simulink model "sampleModel123"  (Simulink 9.1)
settings: Solver=VariableStepAuto  StartTime=0.0  StopTime=10.0  RelTol=1e-3
undefined symbols (not defined in the file): DiscIntNeverNeededParam, Newton, Raphson
libraries: simulink x12
settings Model: SuppressorTable="22 serialization::archive 11 0 6 0 0 1 8 0 0 0 0 6 0 0 1 0 22 sampleModel123/cfblk32 0 6 0 0 2 8 0 0 0 0 6 41 Simulink:DataType:WarningOverFlowDetected 0 0 0 6 0  0  0 0 0 0 8 20160523 0 0 0 10 57 55 0 1 40 SimulinkFixedPoint:util:Overflowoccurred 0 0 0  0  8 20160523 0 10 57 55 0 1"  Creator=DELL  LastModifiedBy=DELL
settings DataIOCC: SaveFormat=Dataset
settings OptimizationCC: LifeSpan=auto
settings DebuggingCC: UnderspecifiedInitializationDetection=Simplified  MergeDetectMultiDrivingBlocksExec=error  SFUnexpectedBacktrackingDiag=error  SFNoUnconditionalDefaultTransitionDiag=error  SFExecutionAtInitializationDiag=warning
settings HardwareCC: ProdBitPerPointer=64  ProdBitPerSizeT=64  ProdBitPerPtrDiffT=64  ProdLargestAtomicFloat=Float  ProdIntDivRoundTo=Zero  ProdEndianess=LittleEndian  ProdWordSize=64  ProdHWDeviceType=Intel->x86-64 (Windows64)
settings ModelReferenceCC: PropagateSignalLabelsOutOfModel=on
settings CodeAppCC: StateflowObjectComments=off
settings GRTTargetCC: TargetLangStandard=C99 (ISO)  CombineOutputUpdateFcns=on  GRTInterface=off
settings ConfigComp: CovMetricSettings=dwe  CovHtmlReporting=off  CovSaveCumulativeToWorkspaceVar=off  CovSaveSingleToWorkspaceVar=off  CovExternalEMLEnable=on

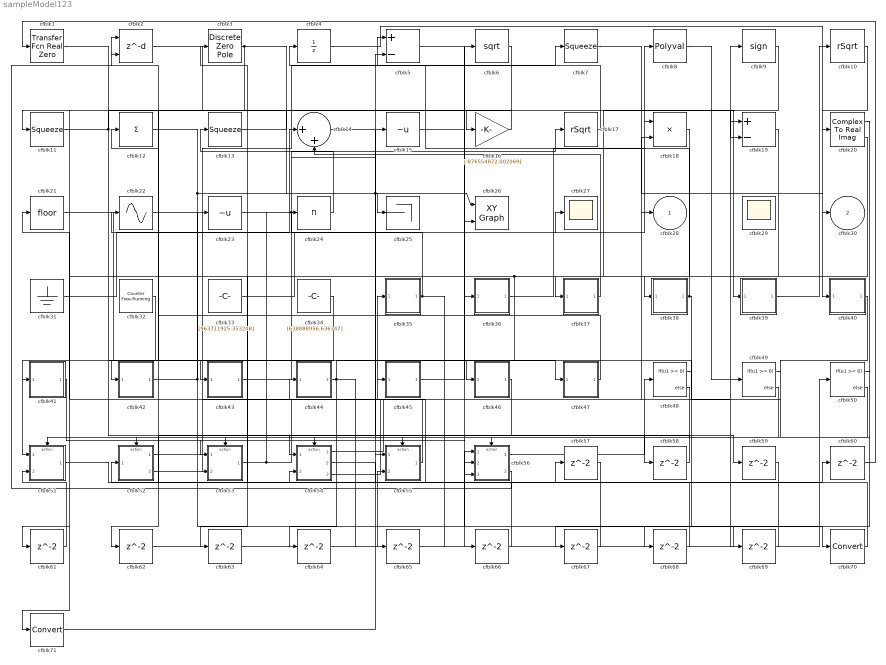
== system sampleModel123 ==
  cfblk1 : simulink/Discrete/Transfer Fcn Real Zero  ZeroZ=0.75  ICPrevInput=0.0  DoSatur=off
      settings: SourceProductName=Simulink  SourceProductBaseCode=SL
  cfblk10 : Sqrt  Operator=rSqrt  AlgorithmType=Newton-Raphson  SaturateOnIntegerOverflow=on
  cfblk11 : Squeeze
  cfblk12 : Sum  Inputs=+
  cfblk13 : Squeeze
  cfblk14 : Sum  Inputs=|++
  cfblk15 : UnaryMinus
  cfblk16 : Gain  Gain=[-876554872.002069]
  cfblk17 : Sqrt  Operator=rSqrt  AlgorithmType=Newton-Raphson  SaturateOnIntegerOverflow=on
  cfblk18 : Product  Inputs=**
  cfblk19 : Sum  Inputs=+-
  cfblk2 : Delay  DelayLengthSource=Input port  SampleTime=1
      settings: InputPortMap=u0,p1
  cfblk20 : ComplexToRealImag
  cfblk21 : Rounding
  cfblk22 : Sin  TimeSource=Use external signal  SampleTime=0
  cfblk23 : UnaryMinus
  cfblk24 : Product  Inputs=*
  cfblk25 : Terminator
  cfblk26 : simulink/Sinks/XY Graph  xmin=-1  xmax=1  ymin=-1  ymax=1  st=-1
  cfblk27 : Scope
  cfblk29 : Scope
      settings: Floating=on
  cfblk3 : DiscreteZeroPole  Poles=[0 0.5]  Gain=1
  cfblk31 : Ground
  cfblk32 : simulink/Sources/Counter Free-Running  NumBits=[29.000000]  tsamp=-1
  cfblk33 : Constant  Value=[963711925.353248]  SampleTime=1
  cfblk34 : Constant  Value=[638888956.636347]  SampleTime=1
  cfblk35 : Subsystem
  cfblk36 : Subsystem
  cfblk37 : Subsystem
  cfblk38 : Subsystem
  cfblk39 : Subsystem
  cfblk4 : UnitDelay
  cfblk40 : Subsystem
  cfblk41 : Subsystem
  cfblk42 : Subsystem
  cfblk43 : Subsystem
  cfblk44 : Subsystem
  cfblk45 : Subsystem
  cfblk46 : Subsystem
  cfblk47 : Subsystem
  cfblk48 : If  IfExpression=u1 >= 0  SampleTime=1
  cfblk49 : If  IfExpression=u1 >= 0  SampleTime=1
  cfblk5 : Sum  Inputs=+-
  cfblk50 : If  IfExpression=u1 >= 0  SampleTime=1
  cfblk51 : Subsystem  TreatAsAtomicUnit=on
  cfblk52 : Subsystem  TreatAsAtomicUnit=on
  cfblk53 : Subsystem  TreatAsAtomicUnit=on
  cfblk54 : Subsystem  TreatAsAtomicUnit=on
  cfblk55 : Subsystem  TreatAsAtomicUnit=on
  cfblk56 : Subsystem  TreatAsAtomicUnit=on
  cfblk{57..69} (13 alike) : Delay  SampleTime=1
  cfblk6 : Sqrt  SaturateOnIntegerOverflow=on
  cfblk7 : Squeeze
  cfblk70 : DataTypeConversion
  cfblk71 : DataTypeConversion
  cfblk8 : Polyval  Coefs=[ +2.081618890e-019, -1.441693666e-014, +4.719686976e-010, -8.536869453e-006, +1.621573104e-001, -8.087801117e+001 ]
  cfblk9 : Signum
  cfblk28 : Outport
  cfblk30 : Outport  Port=2
  wires:
  cfblk24/1 -> cfblk13/1
  cfblk16/1 -> cfblk11/1
  cfblk23/1 -> cfblk8/1, cfblk5/2
  cfblk4/1 -> cfblk40/1(cfblk1)
  cfblk10/1 -> cfblk20/1
  cfblk34/1 -> cfblk51/1(cfblk1)
  cfblk8/1 -> cfblk49/1
  cfblk43/1(cfblk2) -> cfblk17/1
  cfblk56/1(cfblk2) -> cfblk48/1
  cfblk52/1(cfblk2) -> cfblk7/1
  cfblk40/1(cfblk2) -> cfblk44/1(cfblk1)
  cfblk12/1 -> cfblk26/1, cfblk56/3(cfblk8)
  cfblk6/1 -> cfblk41/1(cfblk1)
  cfblk17/1 -> cfblk4/1
  cfblk14/1 -> cfblk26/2, cfblk59/1
  cfblk39/1(cfblk2) -> cfblk10/1
  cfblk9/1 -> cfblk37/1(cfblk1)
  cfblk36/1(cfblk2) -> cfblk18/1
  cfblk56/2(cfblk9) -> cfblk2/1
  cfblk31/1 -> cfblk14/1
  cfblk21/1 -> cfblk43/1(cfblk1)
  cfblk13/1 -> cfblk16/1
  cfblk55/1(cfblk2) -> cfblk21/1
  cfblk5/1 -> cfblk36/1(cfblk1)
  cfblk35/1(cfblk2) -> cfblk22/1, cfblk66/1
  cfblk52/2(cfblk16) -> cfblk35/1(cfblk1)
  cfblk37/1(cfblk2) -> cfblk14/2
  cfblk7/1 -> cfblk30/1
  cfblk54/1(cfblk2) -> cfblk9/1
  cfblk41/1(cfblk2) -> cfblk53/1(cfblk1)
  cfblk2/1 -> cfblk39/1(cfblk1)
  cfblk53/1(cfblk2) -> cfblk28/1, cfblk24/1
  cfblk22/1 -> cfblk53/2(cfblk10)
  cfblk33/1 -> cfblk6/1
  cfblk19/1 -> cfblk46/1(cfblk1), cfblk63/1
  cfblk38/1(cfblk2) -> cfblk5/1, cfblk68/1
  cfblk47/1(cfblk2) -> cfblk12/1
  cfblk44/1(cfblk2) -> cfblk64/1, cfblk65/1
  cfblk42/1(cfblk2) -> cfblk23/1, cfblk69/1
  cfblk45/1(cfblk2) -> cfblk27/1
  cfblk20/2 -> cfblk38/1(cfblk1)
  cfblk3/1 -> cfblk25/1, cfblk42/1(cfblk1)
  cfblk1/1 -> cfblk47/1(cfblk1)
  cfblk11/1 -> cfblk19/2, cfblk58/1
  cfblk54/3(cfblk16) -> cfblk18/2
  cfblk48/1 -> cfblk51/Action
  cfblk48/2 -> cfblk52/Action
  cfblk49/1 -> cfblk53/Action
  cfblk49/2 -> cfblk54/Action
  cfblk50/1 -> cfblk55/Action
  cfblk50/2 -> cfblk56/Action
  cfblk51/1(cfblk2) -> cfblk57/1
  cfblk57/1 -> cfblk56/2(cfblk7)
  cfblk58/1 -> cfblk54/1(cfblk1)
  cfblk59/1 -> cfblk54/2(cfblk14)
  cfblk54/2(cfblk15) -> cfblk60/1
  cfblk60/1 -> cfblk1/1
  cfblk18/1 -> cfblk61/1
  cfblk61/1 -> cfblk51/2(cfblk8)
  cfblk46/1(cfblk2) -> cfblk62/1
  cfblk62/1 -> cfblk56/1(cfblk1)
  cfblk63/1 -> cfblk55/2(cfblk8)
  cfblk64/1 -> cfblk19/1
  cfblk65/1 -> cfblk50/1
  cfblk66/1 -> cfblk52/1(cfblk1)
  cfblk20/1 -> cfblk67/1
  cfblk67/1 -> cfblk2/2
  cfblk68/1 -> cfblk55/1(cfblk1)
  cfblk69/1 -> cfblk3/1
  cfblk15/1 -> cfblk70/1
  cfblk70/1 -> cfblk45/1(cfblk1)
  cfblk32/1 -> cfblk71/1
  cfblk71/1 -> cfblk15/1

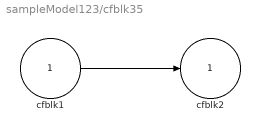
== system sampleModel123/cfblk35 ==
  cfblk1 : Inport
  cfblk2 : Outport
  wires:
  cfblk1/1 -> cfblk2/1

== system sampleModel123/cfblk36 ==
  cfblk1 : Inport
  cfblk2 : Outport
  wires:
  cfblk1/1 -> cfblk2/1

== system sampleModel123/cfblk37 ==
  cfblk1 : Inport
  cfblk2 : Outport
  wires:
  cfblk1/1 -> cfblk2/1

== system sampleModel123/cfblk38 ==
  cfblk1 : Inport
  cfblk2 : Outport
  wires:
  cfblk1/1 -> cfblk2/1

== system sampleModel123/cfblk39 ==
  cfblk1 : Inport
  cfblk2 : Outport
  wires:
  cfblk1/1 -> cfblk2/1

== system sampleModel123/cfblk40 ==
  cfblk1 : Inport
  cfblk2 : Outport
  wires:
  cfblk1/1 -> cfblk2/1

== system sampleModel123/cfblk41 ==
  cfblk1 : Inport
  cfblk2 : Outport
  wires:
  cfblk1/1 -> cfblk2/1

== system sampleModel123/cfblk42 ==
  cfblk1 : Inport
  cfblk2 : Outport
  wires:
  cfblk1/1 -> cfblk2/1

== system sampleModel123/cfblk43 ==
  cfblk1 : Inport
  cfblk2 : Outport
  wires:
  cfblk1/1 -> cfblk2/1

== system sampleModel123/cfblk44 ==
  cfblk1 : Inport
  cfblk2 : Outport
  wires:
  cfblk1/1 -> cfblk2/1

== system sampleModel123/cfblk45 ==
  cfblk1 : Inport
  cfblk2 : Outport
  wires:
  cfblk1/1 -> cfblk2/1

== system sampleModel123/cfblk46 ==
  cfblk1 : Inport
  cfblk2 : Outport
  wires:
  cfblk1/1 -> cfblk2/1

== system sampleModel123/cfblk47 ==
  cfblk1 : Inport
  cfblk2 : Outport
  wires:
  cfblk1/1 -> cfblk2/1

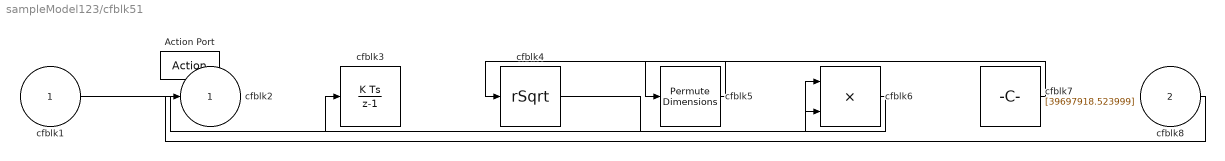
== system sampleModel123/cfblk51 ==
  cfblk1 : Inport
  cfblk8 : Inport  Port=2
  Action Port : ActionPort  ActionType=then
  cfblk3 : DiscreteIntegrator  SampleTime=-1  ICPrevOutput=DiscIntNeverNeededParam  ICPrevScaledInput=DiscIntNeverNeededParam
  cfblk4 : Sqrt  Operator=rSqrt  AlgorithmType=Newton-Raphson  SaturateOnIntegerOverflow=on
  cfblk5 : PermuteDimensions
  cfblk6 : Product  Inputs=**
  cfblk7 : Constant  Value=[39697918.523999]  SampleTime=1
  cfblk2 : Outport
  wires:
  cfblk7/1 -> cfblk5/1
  cfblk6/1 -> cfblk3/1
  cfblk1/1 -> cfblk6/1
  cfblk5/1 -> cfblk4/1
  cfblk8/1 -> cfblk2/1
  cfblk4/1 -> cfblk6/2

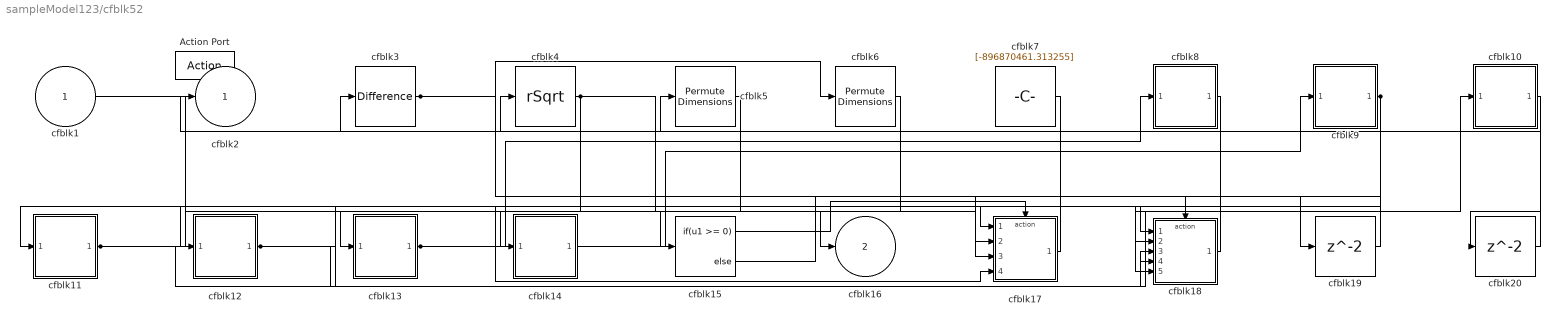
== system sampleModel123/cfblk52 ==
  cfblk1 : Inport
  Action Port : ActionPort  ActionType=else
  cfblk10 : Subsystem
  cfblk11 : Subsystem
  cfblk12 : Subsystem
  cfblk13 : Subsystem
  cfblk14 : Subsystem
  cfblk15 : If  IfExpression=u1 >= 0  SampleTime=1
  cfblk17 : Subsystem  TreatAsAtomicUnit=on
  cfblk18 : Subsystem  TreatAsAtomicUnit=on
  cfblk19 : Delay
  cfblk20 : Delay
  cfblk3 : simulink/Discrete/Difference  ICPrevInput=0.0  OutMin=[]  OutMax=[]  OutDataTypeStr=Inherit: Inherit via back propagation  OutDataType=fixdt(1, 16)  OutScaling=2^-10  DoSatur=off
  cfblk4 : Sqrt  Operator=rSqrt  AlgorithmType=Newton-Raphson  SaturateOnIntegerOverflow=on
  cfblk5 : PermuteDimensions
  cfblk6 : PermuteDimensions
  cfblk7 : Constant  Value=[-896870461.313255]  SampleTime=1
  cfblk8 : Subsystem
  cfblk9 : Subsystem
  cfblk2 : Outport
  cfblk16 : Outport  Port=2
  wires:
  cfblk11/1(cfblk2) -> cfblk5/1, cfblk18/4(cfblk16)
  cfblk13/1(cfblk2) -> cfblk8/1(cfblk1), cfblk18/2(cfblk14), cfblk17/4(cfblk10)
  cfblk14/1(cfblk2) -> cfblk9/1(cfblk1)
  cfblk6/1 -> cfblk16/1
  cfblk4/1 -> cfblk13/1(cfblk1), cfblk17/3(cfblk9)
  cfblk8/1(cfblk2) -> cfblk12/1(cfblk1)
  cfblk3/1 -> cfblk6/1, cfblk19/1
  cfblk5/1 -> cfblk14/1(cfblk1)
  cfblk1/1 -> cfblk15/1
  cfblk7/1 -> cfblk11/1(cfblk1)
  cfblk12/1(cfblk2) -> cfblk10/1(cfblk1), cfblk18/1(cfblk1), cfblk18/3(cfblk15)
  cfblk18/1(cfblk2) -> cfblk2/1
  cfblk9/1(cfblk2) -> cfblk17/1(cfblk1), cfblk18/5(cfblk17)
  cfblk17/1(cfblk2) -> cfblk3/1
  cfblk15/1 -> cfblk17/Action
  cfblk15/2 -> cfblk18/Action
  cfblk19/1 -> cfblk17/2(cfblk8)
  cfblk10/1(cfblk2) -> cfblk20/1
  cfblk20/1 -> cfblk4/1

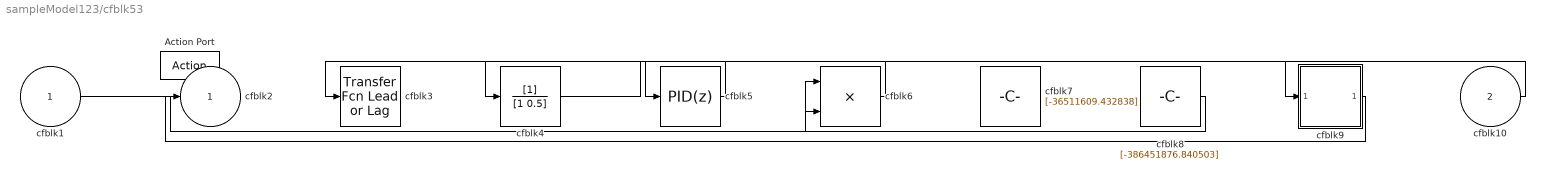
== system sampleModel123/cfblk53 ==
  cfblk1 : Inport
  cfblk10 : Inport  Port=2
  Action Port : ActionPort  ActionType=then
  cfblk3 : simulink/Discrete/Transfer Fcn Lead or Lag  PoleZ=0.95  ZeroZ=0.75  ICPrevOutput=0.0  ICPrevInput=0.0  DoSatur=off
      settings: SourceProductName=Simulink  SourceProductBaseCode=SL
  cfblk4 : DiscreteFilter
  cfblk5 : simulink/Continuous/PID Controller  Controller=PID  TimeDomain=Discrete-time  SampleTime=-1  IntegratorMethod=Forward Euler  FilterMethod=Forward Euler  Form=Parallel  UseFilter=on  ControllerParametersSource=internal  P=1  I=1  D=0  N=100  InitialConditionSource=internal  InitialConditionForIntegrator=0  InitialConditionForFilter=0  ExternalReset=none  LimitOutput=off  UpperSaturationLimit=inf  LowerSaturationLimit=-inf  LinearizeAsGain=off  AntiWindupMode=none  Kb=1  TrackingMode=off  Kt=1  PParamMin=[]  PParamMax=[]  IParamMin=[]  IParamMax=[]  DParamMin=[]  DParamMax=[]  NParamMin=[]  NParamMax=[]  KbParamMin=[]  KbParamMax=[]  KtParamMin=[]  KtParamMax=[]  POutMin=[]  POutMax=[]  IOutMin=[]  IOutMax=[]  DOutMin=[]  DOutMax=[]  NOutMin=[]  NOutMax=[]  KbOutMin=[]  KbOutMax=[]  KtOutMin=[]  KtOutMax=[]  IntegratorOutMin=[]  IntegratorOutMax=[]  FilterOutMin=[]  FilterOutMax=[]  SumOutMin=[]  SumOutMax=[]  SumI1OutMin=[]  SumI1OutMax=[]  SumI2OutMin=[]  SumI2OutMax=[]  SumI3OutMin=[]  SumI3OutMax=[]  SumDOutMin=[]  SumDOutMax=[]  SaturationOutMin=[]  SaturationOutMax=[]  IntegratorContinuousStateAttributes=''  IntegratorStateMustResolveToSignalObject=off  IntegratorRTWStateStorageClass=Auto  FilterContinuousStateAttributes=''  FilterStateMustResolveToSignalObject=off  FilterRTWStateStorageClass=Auto  DifferentiatorICPrevScaledInput=0  DifferentiatorOutMin=[]  DifferentiatorOutMax=[]  FilterDiffOutCoefMin=[]  FilterDiffOutCoefMax=[]  SumDenOutMin=[]  SumDenOutMax=[]  SumNumOutMin=[]  SumNumOutMax=[]  ReciprocalOutMin=[]  ReciprocalOutMax=[]  DivideOutMin=[]  DivideOutMax=[]  TunerSelectOption=Transfer Function Based (PID Tuner App)
  cfblk6 : Product
  cfblk7 : Constant  Value=[-36511609.432838]  SampleTime=1
  cfblk8 : Constant  Value=[-386451876.840503]  SampleTime=1
  cfblk9 : Subsystem
  cfblk2 : Outport
  wires:
  cfblk10/1 -> cfblk3/1
  cfblk1/1 -> cfblk6/1
  cfblk8/1 -> cfblk6/2
  cfblk6/1 -> cfblk5/1
  cfblk9/1(cfblk2) -> cfblk2/1
  cfblk4/1 -> cfblk9/1(cfblk1)
  cfblk5/1 -> cfblk4/1

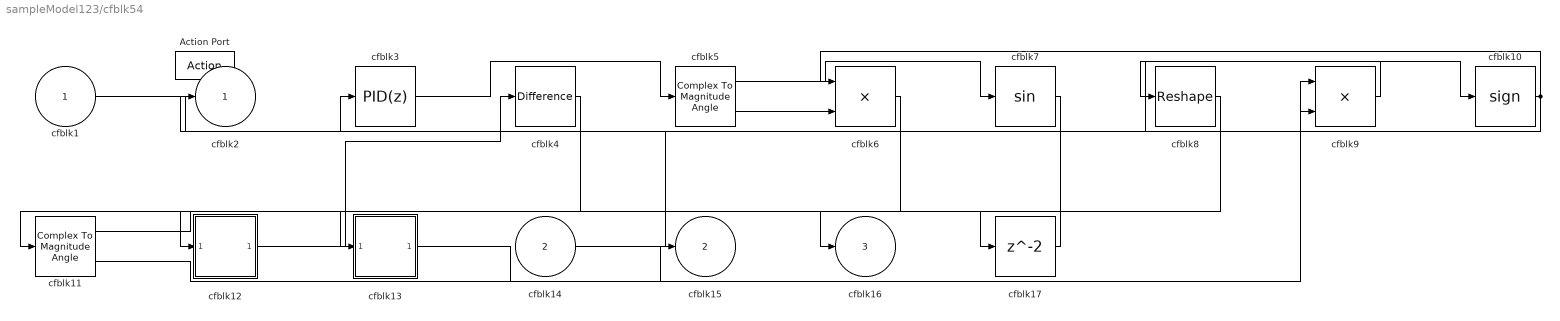
== system sampleModel123/cfblk54 ==
  cfblk1 : Inport
  cfblk14 : Inport  Port=2
  Action Port : ActionPort  ActionType=else
  cfblk10 : Signum
  cfblk11 : ComplexToMagnitudeAngle
  cfblk12 : Subsystem
  cfblk13 : Subsystem
  cfblk17 : Delay
  cfblk3 : simulink/Continuous/PID Controller  Controller=PID  TimeDomain=Discrete-time  SampleTime=-1  IntegratorMethod=Forward Euler  FilterMethod=Forward Euler  Form=Parallel  UseFilter=on  ControllerParametersSource=internal  P=1  I=1  D=0  N=100  InitialConditionSource=internal  InitialConditionForIntegrator=0  InitialConditionForFilter=0  ExternalReset=none  LimitOutput=off  UpperSaturationLimit=inf  LowerSaturationLimit=-inf  LinearizeAsGain=off  AntiWindupMode=none  Kb=1  TrackingMode=off  Kt=1  PParamMin=[]  PParamMax=[]  IParamMin=[]  IParamMax=[]  DParamMin=[]  DParamMax=[]  NParamMin=[]  NParamMax=[]  KbParamMin=[]  KbParamMax=[]  KtParamMin=[]  KtParamMax=[]  POutMin=[]  POutMax=[]  IOutMin=[]  IOutMax=[]  DOutMin=[]  DOutMax=[]  NOutMin=[]  NOutMax=[]  KbOutMin=[]  KbOutMax=[]  KtOutMin=[]  KtOutMax=[]  IntegratorOutMin=[]  IntegratorOutMax=[]  FilterOutMin=[]  FilterOutMax=[]  SumOutMin=[]  SumOutMax=[]  SumI1OutMin=[]  SumI1OutMax=[]  SumI2OutMin=[]  SumI2OutMax=[]  SumI3OutMin=[]  SumI3OutMax=[]  SumDOutMin=[]  SumDOutMax=[]  SaturationOutMin=[]  SaturationOutMax=[]  IntegratorContinuousStateAttributes=''  IntegratorStateMustResolveToSignalObject=off  IntegratorRTWStateStorageClass=Auto  FilterContinuousStateAttributes=''  FilterStateMustResolveToSignalObject=off  FilterRTWStateStorageClass=Auto  DifferentiatorICPrevScaledInput=0  DifferentiatorOutMin=[]  DifferentiatorOutMax=[]  FilterDiffOutCoefMin=[]  FilterDiffOutCoefMax=[]  SumDenOutMin=[]  SumDenOutMax=[]  SumNumOutMin=[]  SumNumOutMax=[]  ReciprocalOutMin=[]  ReciprocalOutMax=[]  DivideOutMin=[]  DivideOutMax=[]  TunerSelectOption=Transfer Function Based (PID Tuner App)
  cfblk4 : simulink/Discrete/Difference  ICPrevInput=0.0  OutMin=[]  OutMax=[]  OutDataTypeStr=Inherit: Inherit via back propagation  OutDataType=fixdt(1, 16)  OutScaling=2^-10  DoSatur=off
  cfblk5 : ComplexToMagnitudeAngle
  cfblk6 : Product
  cfblk7 : Trigonometry
  cfblk8 : Reshape
  cfblk9 : Product
  cfblk2 : Outport
  cfblk15 : Outport  Port=2
  cfblk16 : Outport  Port=3
  wires:
  cfblk8/1 -> cfblk16/1
  cfblk12/1(cfblk2) -> cfblk4/1
  cfblk5/1 -> cfblk7/1
  cfblk3/1 -> cfblk5/1
  cfblk14/1 -> cfblk10/1
  cfblk13/1(cfblk2) -> cfblk9/1
  cfblk11/2 -> cfblk15/1
  cfblk1/1 -> cfblk9/2
  cfblk4/1 -> cfblk13/1(cfblk1)
  cfblk6/1 -> cfblk11/1
  cfblk7/1 -> cfblk12/1(cfblk1)
  cfblk10/1 -> cfblk6/1, cfblk2/1
  cfblk9/1 -> cfblk8/1
  cfblk5/2 -> cfblk6/2
  cfblk11/1 -> cfblk17/1
  cfblk17/1 -> cfblk3/1

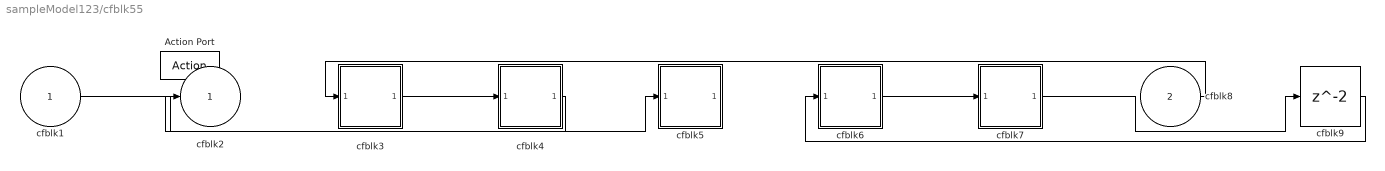
== system sampleModel123/cfblk55 ==
  cfblk1 : Inport
  cfblk8 : Inport  Port=2
  Action Port : ActionPort  ActionType=then
  cfblk3 : Subsystem
  cfblk4 : Subsystem
  cfblk5 : Subsystem
  cfblk6 : Subsystem
  cfblk7 : Subsystem
  cfblk9 : Delay
  cfblk2 : Outport
  wires:
  cfblk6/1(cfblk2) -> cfblk7/1(cfblk1)
  cfblk1/1 -> cfblk5/1(cfblk1)
  cfblk8/1 -> cfblk3/1(cfblk1)
  cfblk3/1(cfblk2) -> cfblk4/1(cfblk1)
  cfblk4/1(cfblk2) -> cfblk2/1
  cfblk7/1(cfblk2) -> cfblk9/1
  cfblk9/1 -> cfblk6/1(cfblk1)

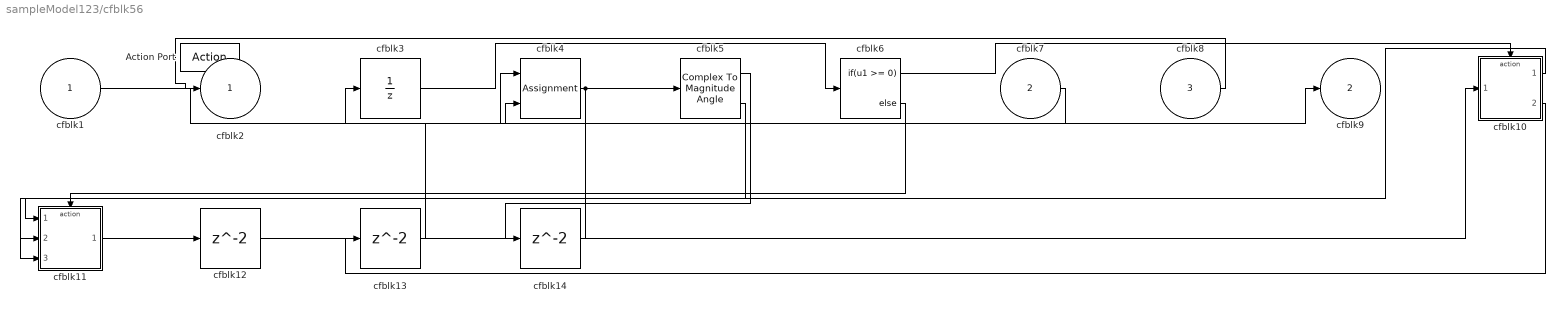
== system sampleModel123/cfblk56 ==
  cfblk1 : Inport
  cfblk7 : Inport  Port=2
  cfblk8 : Inport  Port=3
  Action Port : ActionPort  ActionType=else
  cfblk10 : Subsystem  TreatAsAtomicUnit=on
  cfblk11 : Subsystem  TreatAsAtomicUnit=on
  cfblk12 : Delay
  cfblk13 : Delay
  cfblk14 : Delay
  cfblk3 : UnitDelay  SampleTime=-1
  cfblk4 : Assignment  DiagnosticForDimensions=Warning  IndexOptions=Index vector (dialog)  Indices=1  OutputSizes=1
  cfblk5 : ComplexToMagnitudeAngle
  cfblk6 : If  IfExpression=u1 >= 0  SampleTime=1
  cfblk2 : Outport
  cfblk9 : Outport  Port=2
  wires:
  cfblk1/1 -> cfblk9/1
  cfblk8/1 -> cfblk2/1
  cfblk3/1 -> cfblk6/1
  cfblk10/1(cfblk2) -> cfblk11/1(cfblk1)
  cfblk7/1 -> cfblk4/2
  cfblk4/1 -> cfblk11/2(cfblk9), cfblk5/1
  cfblk5/2 -> cfblk11/3(cfblk10)
  cfblk6/1 -> cfblk10/Action
  cfblk6/2 -> cfblk11/Action
  cfblk11/1(cfblk2) -> cfblk12/1
  cfblk12/1 -> cfblk10/1(cfblk1)
  cfblk10/2(cfblk16) -> cfblk13/1
  cfblk13/1 -> cfblk3/1
  cfblk5/1 -> cfblk14/1
  cfblk14/1 -> cfblk4/1

== system sampleModel123/cfblk52/cfblk10 ==
  cfblk1 : Inport
  cfblk2 : Outport
  wires:
  cfblk1/1 -> cfblk2/1

== system sampleModel123/cfblk52/cfblk11 ==
  cfblk1 : Inport
  cfblk2 : Outport
  wires:
  cfblk1/1 -> cfblk2/1

== system sampleModel123/cfblk52/cfblk12 ==
  cfblk1 : Inport
  cfblk2 : Outport
  wires:
  cfblk1/1 -> cfblk2/1

== system sampleModel123/cfblk52/cfblk13 ==
  cfblk1 : Inport
  cfblk2 : Outport
  wires:
  cfblk1/1 -> cfblk2/1

== system sampleModel123/cfblk52/cfblk14 ==
  cfblk1 : Inport
  cfblk2 : Outport
  wires:
  cfblk1/1 -> cfblk2/1

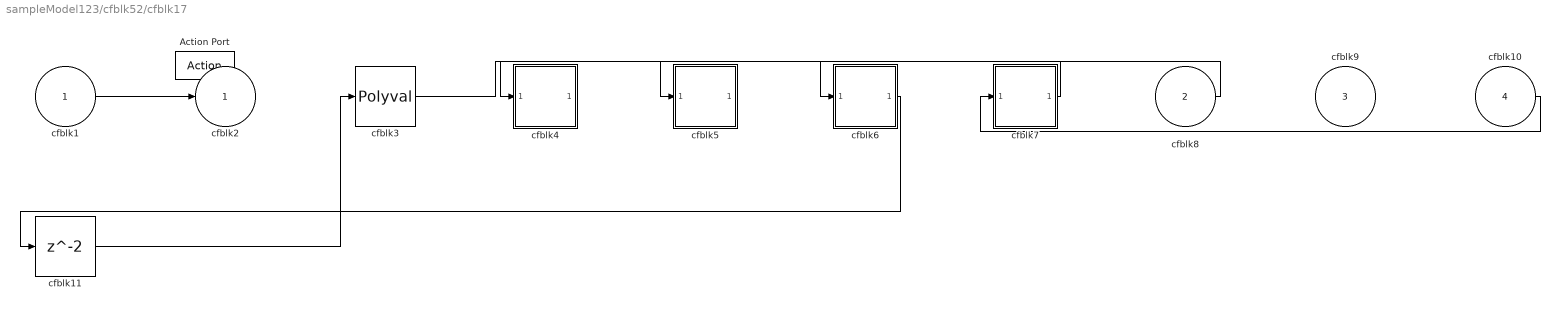
== system sampleModel123/cfblk52/cfblk17 ==
  cfblk1 : Inport
  cfblk8 : Inport  Port=2
  cfblk9 : Inport  Port=3
  cfblk10 : Inport  Port=4
  Action Port : ActionPort  ActionType=then
  cfblk11 : Delay
  cfblk3 : Polyval  Coefs=[ +2.081618890e-019, -1.441693666e-014, +4.719686976e-010, -8.536869453e-006, +1.621573104e-001, -8.087801117e+001 ]
  cfblk4 : Subsystem
  cfblk5 : Subsystem
  cfblk6 : Subsystem
  cfblk7 : Subsystem
  cfblk2 : Outport
  wires:
  cfblk7/1(cfblk2) -> cfblk4/1(cfblk1)
  cfblk10/1 -> cfblk7/1(cfblk1)
  cfblk1/1 -> cfblk2/1
  cfblk8/1 -> cfblk5/1(cfblk1)
  cfblk3/1 -> cfblk6/1(cfblk1)
  cfblk6/1(cfblk2) -> cfblk11/1
  cfblk11/1 -> cfblk3/1

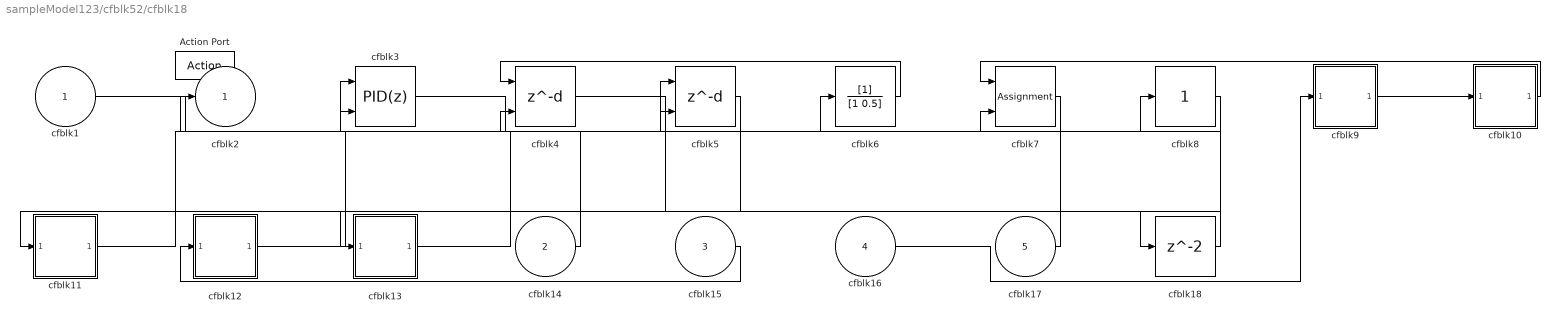
== system sampleModel123/cfblk52/cfblk18 ==
  cfblk1 : Inport
  cfblk14 : Inport  Port=2
  cfblk15 : Inport  Port=3
  cfblk16 : Inport  Port=4
  cfblk17 : Inport  Port=5
  Action Port : ActionPort  ActionType=else
  cfblk10 : Subsystem
  cfblk11 : Subsystem
  cfblk12 : Subsystem
  cfblk13 : Subsystem
  cfblk18 : Delay
  cfblk3 : simulink/Continuous/PID Controller (2DOF)  Controller=PID  TimeDomain=Discrete-time  SampleTime=-1  IntegratorMethod=Forward Euler  FilterMethod=Forward Euler  Form=Parallel  UseFilter=on  ControllerParametersSource=internal  P=1  I=1  D=0  N=100  b=1  c=1  InitialConditionSource=internal  InitialConditionForIntegrator=0  InitialConditionForFilter=0  ExternalReset=none  LimitOutput=off  UpperSaturationLimit=inf  LowerSaturationLimit=-inf  LinearizeAsGain=off  AntiWindupMode=none  Kb=1  TrackingMode=off  Kt=1  PParamMin=[]  PParamMax=[]  IParamMin=[]  IParamMax=[]  DParamMin=[]  DParamMax=[]  NParamMin=[]  NParamMax=[]  bParamMin=[]  bParamMax=[]  cParamMin=[]  cParamMax=[]  KbParamMin=[]  KbParamMax=[]  KtParamMin=[]  KtParamMax=[]  POutMin=[]  POutMax=[]  IOutMin=[]  IOutMax=[]  DOutMin=[]  DOutMax=[]  NOutMin=[]  NOutMax=[]  bOutMin=[]  bOutMax=[]  cOutMin=[]  cOutMax=[]  KbOutMin=[]  KbOutMax=[]  KtOutMin=[]  KtOutMax=[]  IntegratorOutMin=[]  IntegratorOutMax=[]  FilterOutMin=[]  FilterOutMax=[]  SumOutMin=[]  SumOutMax=[]  Sum1OutMin=[]  Sum1OutMax=[]  Sum2OutMin=[]  Sum2OutMax=[]  Sum3OutMin=[]  Sum3OutMax=[]  SumI1OutMin=[]  SumI1OutMax=[]  SumI2OutMin=[]  SumI2OutMax=[]  SumI3OutMin=[]  SumI3OutMax=[]  SumDOutMin=[]  SumDOutMax=[]  SaturationOutMin=[]  SaturationOutMax=[]  IntegratorContinuousStateAttributes=''  IntegratorStateMustResolveToSignalObject=off  IntegratorRTWStateStorageClass=Auto  FilterContinuousStateAttributes=''  FilterStateMustResolveToSignalObject=off  FilterRTWStateStorageClass=Auto  DifferentiatorICPrevScaledInput=0  DifferentiatorOutMin=[]  DifferentiatorOutMax=[]  FilterDiffOutCoefMin=[]  FilterDiffOutCoefMax=[]  SumDenOutMin=[]  SumDenOutMax=[]  SumNumOutMin=[]  SumNumOutMax=[]  ReciprocalOutMin=[]  ReciprocalOutMax=[]  DivideOutMin=[]  DivideOutMax=[]  TunerSelectOption=Transfer Function Based (PID Tuner App)
  cfblk4 : Delay  DelayLengthSource=Input port
      settings: InputPortMap=u0,p1
  cfblk5 : Delay  DelayLengthSource=Input port
      settings: InputPortMap=u0,p1
  cfblk6 : DiscreteFilter
  cfblk7 : Assignment  DiagnosticForDimensions=Warning  IndexOptions=Index vector (dialog)  Indices=1  OutputSizes=1
  cfblk8 : simulink/Math Operations/Slider Gain  gain=1  low=0  high=2
  cfblk9 : Subsystem
  cfblk2 : Outport
  wires:
  cfblk8/1 -> cfblk11/1(cfblk1)
  cfblk10/1(cfblk2) -> cfblk7/1
  cfblk14/1 -> cfblk3/1
  cfblk13/1(cfblk2) -> cfblk7/2
  cfblk6/1 -> cfblk4/1
  cfblk16/1 -> cfblk9/1(cfblk1)
  cfblk3/1 -> cfblk6/1
  cfblk9/1(cfblk2) -> cfblk10/1(cfblk1)
  cfblk1/1 -> cfblk5/1
  cfblk12/1(cfblk2) -> cfblk8/1
  cfblk15/1 -> cfblk12/1(cfblk1)
  cfblk7/1 -> cfblk4/2
  cfblk17/1 -> cfblk2/1
  cfblk5/1 -> cfblk13/1(cfblk1)
  cfblk11/1(cfblk2) -> cfblk3/2
  cfblk4/1 -> cfblk18/1
  cfblk18/1 -> cfblk5/2

== system sampleModel123/cfblk52/cfblk8 ==
  cfblk1 : Inport
  cfblk2 : Outport
  wires:
  cfblk1/1 -> cfblk2/1

== system sampleModel123/cfblk52/cfblk9 ==
  cfblk1 : Inport
  cfblk2 : Outport
  wires:
  cfblk1/1 -> cfblk2/1

== system sampleModel123/cfblk53/cfblk9 ==
  cfblk1 : Inport
  cfblk2 : Outport
  wires:
  cfblk1/1 -> cfblk2/1

== system sampleModel123/cfblk54/cfblk12 ==
  cfblk1 : Inport
  cfblk2 : Outport
  wires:
  cfblk1/1 -> cfblk2/1

== system sampleModel123/cfblk54/cfblk13 ==
  cfblk1 : Inport
  cfblk2 : Outport
  wires:
  cfblk1/1 -> cfblk2/1

== system sampleModel123/cfblk55/cfblk3 ==
  cfblk1 : Inport
  cfblk2 : Outport
  wires:
  cfblk1/1 -> cfblk2/1

== system sampleModel123/cfblk55/cfblk4 ==
  cfblk1 : Inport
  cfblk2 : Outport
  wires:
  cfblk1/1 -> cfblk2/1

== system sampleModel123/cfblk55/cfblk5 ==
  cfblk1 : Inport
  cfblk2 : Outport
  wires:
  cfblk1/1 -> cfblk2/1

== system sampleModel123/cfblk55/cfblk6 ==
  cfblk1 : Inport
  cfblk2 : Outport
  wires:
  cfblk1/1 -> cfblk2/1

== system sampleModel123/cfblk55/cfblk7 ==
  cfblk1 : Inport
  cfblk2 : Outport
  wires:
  cfblk1/1 -> cfblk2/1

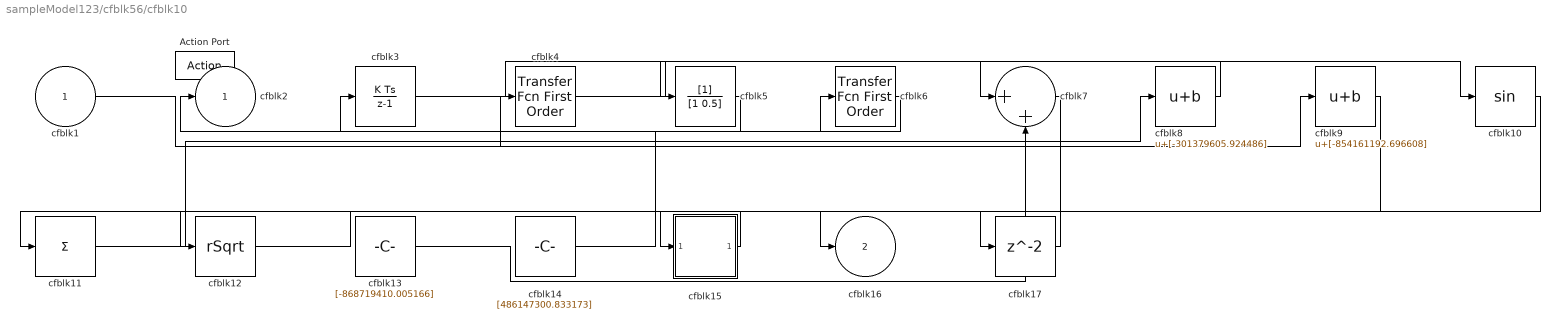
== system sampleModel123/cfblk56/cfblk10 ==
  cfblk1 : Inport
  Action Port : ActionPort  ActionType=then
  cfblk10 : Trigonometry
  cfblk11 : Sum  Inputs=+
  cfblk12 : Sqrt  Operator=rSqrt  AlgorithmType=Newton-Raphson  SaturateOnIntegerOverflow=on
  cfblk13 : Constant  Value=[-868719410.005166]  SampleTime=1
  cfblk14 : Constant  Value=[486147300.833173]  SampleTime=1
  cfblk15 : Subsystem
  cfblk17 : Delay
  cfblk3 : DiscreteIntegrator  SampleTime=-1  ICPrevOutput=DiscIntNeverNeededParam  ICPrevScaledInput=DiscIntNeverNeededParam
  cfblk4 : simulink/Discrete/Transfer Fcn First Order  PoleZ=0.95  ICPrevOutput=0.0  DoSatur=off
      settings: SourceProductName=Simulink
  cfblk5 : DiscreteFilter
  cfblk6 : simulink/Discrete/Transfer Fcn First Order  PoleZ=0.95  ICPrevOutput=0.0  DoSatur=off
      settings: SourceProductName=Simulink
  cfblk7 : Sum  Inputs=|++
  cfblk8 : Bias  Bias=[-301379605.924486]
  cfblk9 : Bias  Bias=[-854161192.696608]
  cfblk2 : Outport
  cfblk16 : Outport  Port=2
  wires:
  cfblk3/1 -> cfblk10/1
  cfblk6/1 -> cfblk3/1
  cfblk4/1 -> cfblk7/1
  cfblk12/1 -> cfblk15/1(cfblk1)
  cfblk11/1 -> cfblk8/1
  cfblk5/1 -> cfblk2/1
  cfblk13/1 -> cfblk7/2
  cfblk15/1(cfblk2) -> cfblk11/1
  cfblk10/1 -> cfblk16/1
  cfblk1/1 -> cfblk9/1
  cfblk8/1 -> cfblk5/1
  cfblk9/1 -> cfblk12/1
  cfblk14/1 -> cfblk6/1
  cfblk7/1 -> cfblk17/1
  cfblk17/1 -> cfblk4/1

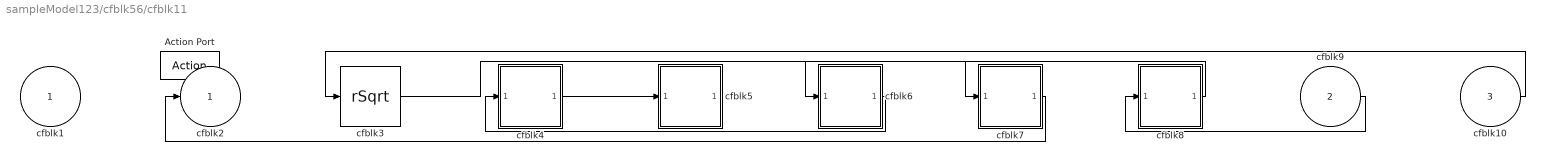
== system sampleModel123/cfblk56/cfblk11 ==
  cfblk1 : Inport
  cfblk9 : Inport  Port=2
  cfblk10 : Inport  Port=3
  Action Port : ActionPort  ActionType=else
  cfblk3 : Sqrt  Operator=rSqrt  AlgorithmType=Newton-Raphson  SaturateOnIntegerOverflow=on
  cfblk4 : Subsystem
  cfblk5 : Subsystem
  cfblk6 : Subsystem
  cfblk7 : Subsystem
  cfblk8 : Subsystem
  cfblk2 : Outport
  wires:
  cfblk4/1(cfblk2) -> cfblk5/1(cfblk1)
  cfblk8/1(cfblk2) -> cfblk6/1(cfblk1)
  cfblk9/1 -> cfblk8/1(cfblk1)
  cfblk10/1 -> cfblk3/1
  cfblk6/1(cfblk2) -> cfblk4/1(cfblk1)
  cfblk7/1(cfblk2) -> cfblk2/1
  cfblk3/1 -> cfblk7/1(cfblk1)

== system sampleModel123/cfblk52/cfblk17/cfblk4 ==
  cfblk1 : Inport
  cfblk2 : Outport
  wires:
  cfblk1/1 -> cfblk2/1

== system sampleModel123/cfblk52/cfblk17/cfblk5 ==
  cfblk1 : Inport
  cfblk2 : Outport
  wires:
  cfblk1/1 -> cfblk2/1

== system sampleModel123/cfblk52/cfblk17/cfblk6 ==
  cfblk1 : Inport
  cfblk2 : Outport
  wires:
  cfblk1/1 -> cfblk2/1

== system sampleModel123/cfblk52/cfblk17/cfblk7 ==
  cfblk1 : Inport
  cfblk2 : Outport
  wires:
  cfblk1/1 -> cfblk2/1

== system sampleModel123/cfblk52/cfblk18/cfblk10 ==
  cfblk1 : Inport
  cfblk2 : Outport
  wires:
  cfblk1/1 -> cfblk2/1

== system sampleModel123/cfblk52/cfblk18/cfblk11 ==
  cfblk1 : Inport
  cfblk2 : Outport
  wires:
  cfblk1/1 -> cfblk2/1

== system sampleModel123/cfblk52/cfblk18/cfblk12 ==
  cfblk1 : Inport
  cfblk2 : Outport
  wires:
  cfblk1/1 -> cfblk2/1

== system sampleModel123/cfblk52/cfblk18/cfblk13 ==
  cfblk1 : Inport
  cfblk2 : Outport
  wires:
  cfblk1/1 -> cfblk2/1

== system sampleModel123/cfblk52/cfblk18/cfblk9 ==
  cfblk1 : Inport
  cfblk2 : Outport
  wires:
  cfblk1/1 -> cfblk2/1

== system sampleModel123/cfblk56/cfblk10/cfblk15 ==
  cfblk1 : Inport
  cfblk2 : Outport
  wires:
  cfblk1/1 -> cfblk2/1

== system sampleModel123/cfblk56/cfblk11/cfblk4 ==
  cfblk1 : Inport
  cfblk2 : Outport
  wires:
  cfblk1/1 -> cfblk2/1

== system sampleModel123/cfblk56/cfblk11/cfblk5 ==
  cfblk1 : Inport
  cfblk2 : Outport
  wires:
  cfblk1/1 -> cfblk2/1

== system sampleModel123/cfblk56/cfblk11/cfblk6 ==
  cfblk1 : Inport
  cfblk2 : Outport
  wires:
  cfblk1/1 -> cfblk2/1

== system sampleModel123/cfblk56/cfblk11/cfblk7 ==
  cfblk1 : Inport
  cfblk2 : Outport
  wires:
  cfblk1/1 -> cfblk2/1

== system sampleModel123/cfblk56/cfblk11/cfblk8 ==
  cfblk1 : Inport
  cfblk2 : Outport
  wires:
  cfblk1/1 -> cfblk2/1
